simulink model "Hybrid_control"  (R2012b)
settings: Solver=ode3  StartTime=0.0  StopTime=inf  FixedStep=0.01  RelTol=1e-3
undefined symbols (not defined in the file or in its folder): HIL
libraries: quarc_library x7, simulink x1
settings Model: SimulationMode=external  ExtModeTrigDuration=5000  Creator=yiwei.liu  LastModifiedBy=yiwei.liu
settings SolverCC: PositivePriorityOrder=on
settings RTWCC: SystemTargetFile=quarc_win64.tlc  TemplateMakefile=quarc_default_tmf  Description=QUARC Win64 Target  ProcessScript=quarc_win64_make_rtw_hook
settings STFCustomTargetCC: TargetPreCompLibLocation=C:\PROGRA~3\QUARC\lib\2012b\win64\release  CodeReplacementLibrary=ANSI_C  GeneratePreprocessorConditionals=Disable all  CombineOutputUpdateFcns=on  GRTInterface=off  SystemTargetFile=quarc_win64.tlc
settings GRTTargetCC: TargetPreCompLibLocation=C:\PROGRA~3\QUARC\lib\2012b\win64\release  ParMdlRefBuildCompliant=off  CompOptLevelCompliant=off  ConcurrentExecutionCompliant=off  MatFileLogging=off  ExtMode=on  ExtModeMexFile=quarc_comm

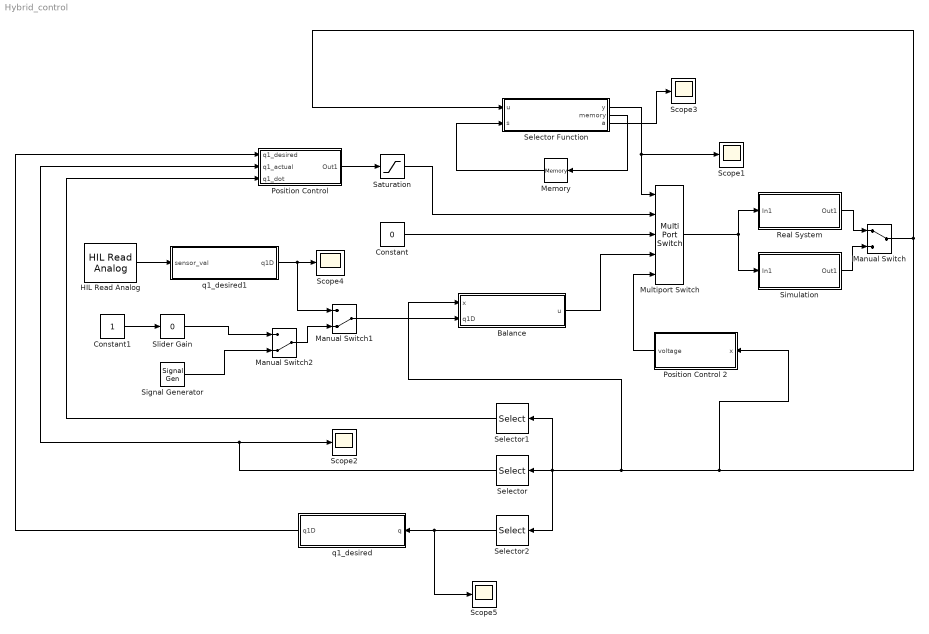
== system Hybrid_control ==
  Balance : MATLAB Function  TreatAsAtomicUnit=on
  Constant : Constant  Value=0
  Constant1 : Constant
  HIL Read Analog : quarc_library/Data Acquisition/Generic/Immediate I//O/HIL Read Analog  object_name=HIL-1  channels=[1]  sample_time=qc_get_step_size  active=on  vector_output=off
  Manual Switch : ManualSwitch
  Manual Switch1 : ManualSwitch  CurrentSetting=0
  Manual Switch2 : ManualSwitch  CurrentSetting=0
  Memory : Memory  X0=4
  Multiport Switch : MultiPortSwitch  Inputs=4
  Position Control : Subsystem  Tag=Simulation  Description=Simulation
  Position Control 2 : Subsystem  Tag=Simulation  Description=Simulation
  Real System : Subsystem
  Saturation : Saturate  UpperLimit=10  LowerLimit=-10
  Scope{1..5} (5 alike) : Scope
      Scope1 settings: TimeRange=10  YMin=3.8  YMax=4.2  SaveName=ScopeData3
      Scope2 settings: SaveName=ScopeData2
      Scope3 settings: YMin=2  YMax=2  SaveName=ScopeData4
      Scope4 settings: TimeRange=10  YMin=-3.5  YMax=5.5  SaveName=ScopeData5
      Scope5 settings: YMin=-12  YMax=9  SaveName=ScopeData6
  Selector : Selector  InputPortWidth=4  IndexOptions=Index vector (dialog)  Indices=[1]  OutputSizes=1
  Selector Function : MATLAB Function  TreatAsAtomicUnit=on
  Selector1 : Selector  InputPortWidth=4  IndexOptions=Index vector (dialog)  Indices=[2]  OutputSizes=1
  Selector2 : Selector  InputPortWidth=4  IndexOptions=Index vector (dialog)  Indices=[3,4]  OutputSizes=1
  Signal Generator : SignalGenerator  Frequency=0.5
  Simulation : Subsystem  Tag=Simulation  Description=Simulation
  Slider Gain : simulink/Math Operations/Slider Gain  low=-3.1416  gain=0  high=3.1416
  q1_desired : MATLAB Function  TreatAsAtomicUnit=on
  q1_desired1 : MATLAB Function  TreatAsAtomicUnit=on
  wires:
  Selector Function/1(y) -> Scope1/1, Multiport Switch/1
  Constant/1 -> Multiport Switch/3
  Selector Function/2(memory) -> Memory/1
  Simulation/1(Out1) -> Manual Switch/2
  Multiport Switch/1 -> Real System/1(In1), Simulation/1(In1)
  Real System/1(Out1) -> Manual Switch/1
  Manual Switch/1 -> Position Control 2/1(x), Balance/1(x), Selector1/1, Selector/1, Selector2/1, Selector Function/1(u)
  Memory/1 -> Selector Function/2(s)
  Position Control/1(Out1) -> Saturation/1
  Selector/1 -> Scope2/1, Position Control/2(q1_actual)
  Balance/1(u) -> Multiport Switch/4
  Selector1/1 -> Position Control/3(q1_dot)
  Selector2/1 -> Scope5/1, q1_desired/1(q)
  q1_desired/1(q1D) -> Position Control/1(q1_desired)
  Saturation/1 -> Multiport Switch/2
  Constant1/1 -> Slider Gain/1
  Position Control 2/1(voltage) -> Multiport Switch/5
  Selector Function/3(a) -> Scope3/1
  HIL Read Analog/1 -> q1_desired1/1(sensor_val)
  q1_desired1/1(q1D) -> Manual Switch1/1, Scope4/1
  Slider Gain/1 -> Manual Switch2/1
  Manual Switch1/1 -> Balance/2(q1D)
  Signal Generator/1 -> Manual Switch2/2
  Manual Switch2/1 -> Manual Switch1/2

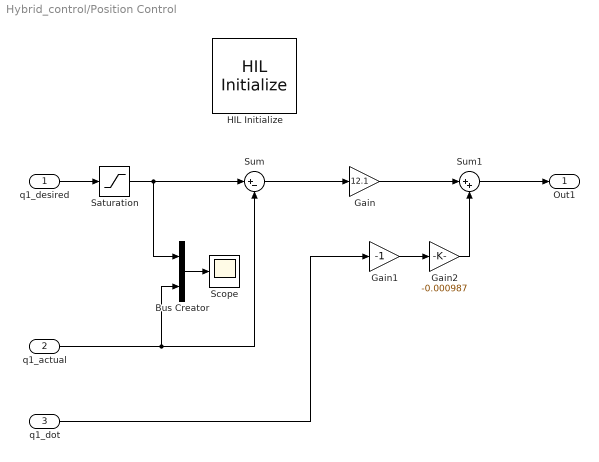
== system Hybrid_control/Position Control ==
  q1_desired : Inport  Description=q1 Desired
  q1_actual : Inport  Port=2
  q1_dot : Inport  Port=3
  Bus Creator : BusCreator  Inputs=2
  Gain : Gain  Gain=12.1
  Gain1 : Gain  Gain=-1
  Gain2 : Gain  Gain=-0.000987
  HIL Initialize : quarc_library/Data Acquisition/Generic/Configuration/HIL Initialize  Priority=-99  object_name=HIL-2  board_type=q2_usb  board_number=0  board_options=d0=digital;d1=digital;led=auto;update_rate=normal;decimation=1  exclusive=off  active=off  hardware_clocks=[0]  clock_modes=[]  initial_clock_frequencies=[]  set_clock_params_at_start=off  set_clock_params_at_switch_in=off  set_clock_frequencies_at_start=off  set_clock_frequencies_at_switch_in=off  analog_input_channels=[0:1]  analog_input_maximums=10  analog_input_minimums=-10  set_analog_input_params_at_start=on  set_analog_input_params_at_switch_in=off  analog_output_channels=[0:1]  analog_output_maximums=10  analog_output_minimums=-10  initial_analog_outputs=[0]  final_analog_outputs=[0]  watchdog_analog_outputs=0  set_analog_output_params_at_start=on  set_analog_output_params_at_switch_in=off  set_analog_outputs_at_start=on  set_analog_outputs_at_switch_in=off  set_analog_outputs_at_terminate=on  set_analog_outputs_at_switch_out=off  set_analog_outputs_on_watchdog=off  digital_input_channels=[]  digital_output_channels=[]  digital_output_configuration=[]  initial_digital_outputs=[1]  final_digital_outputs=[1]  watchdog_digital_outputs=[1]  set_digital_output_params_at_start=off  set_digital_output_params_at_switch_in=off  set_digital_outputs_at_start=on  set_digital_outputs_at_switch_in=off  set_digital_outputs_at_terminate=on  set_digital_outputs_at_switch_out=off  set_digital_outputs_on_watchdog=off  encoder_channels=[0:1]  quadrature=[4]  encoder_filter_frequency=[]  initial_encoder_counts=[0]  set_encoder_params_at_start=on  set_encoder_params_at_switch_in=off  set_encoder_counts_at_start=on  set_encoder_counts_at_switch_in=off  pwm_channels=[]  pwm_modes=[0]  pwm_frequency=1/0.020  pwm_configuration=[]  pwm_alignment=[]  pwm_polarity=[]  pwm_leading_deadband=[]  pwm_trailing_deadband=[]  initial_pwm_outputs=[0]  final_pwm_outputs=[0]  watchdog_pwm_outputs=[0]  set_pwm_params_at_start=on  set_pwm_params_at_switch_in=off  set_pwm_outputs_at_start=on  set_pwm_outputs_at_switch_in=off  set_pwm_outputs_at_terminate=on  set_pwm_outputs_at_switch_out=off  set_pwm_outputs_on_watchdog=off  other_output_channels=[]  initial_other_outputs=[]  final_other_outputs=[]  watchdog_other_outputs=[]  set_other_outputs_at_start=off  set_other_outputs_at_switch_in=off  set_other_outputs_at_terminate=off  set_other_outputs_at_switch_out=off  set_other_outputs_on_watchdog=off
  Saturation : Saturate  UpperLimit=pi/7  LowerLimit=-pi/7
  Scope : Scope
      settings: YMin=0.4  YMax=1.4
  Sum : Sum  Inputs=|+-
  Sum1 : Sum  Inputs=|++
  Out1 : Outport
  wires:
  Gain/1 -> Sum1/1
  Sum/1 -> Gain/1
  Gain1/1 -> Gain2/1
  Gain2/1 -> Sum1/2
  Bus Creator/1 -> Scope/1
  q1_desired/1 -> Saturation/1
  Sum1/1 -> Out1/1
  q1_actual/1 -> Bus Creator/2, Sum/2
  q1_dot/1 -> Gain1/1
  Saturation/1 -> Bus Creator/1, Sum/1

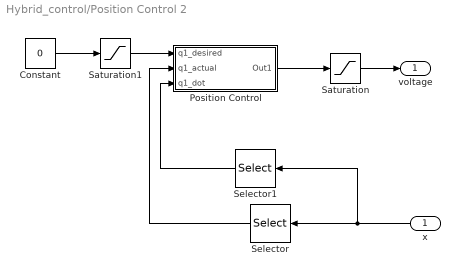
== system Hybrid_control/Position Control 2 ==
  x : Inport  Description=q1 Desired
  Constant : Constant  Value=0
  Position Control : Subsystem  Tag=Simulation  Description=Simulation
  Saturation : Saturate  UpperLimit=2  LowerLimit=-2
  Saturation1 : Saturate  UpperLimit=pi/6  LowerLimit=-pi/6
  Selector : Selector  InputPortWidth=4  IndexOptions=Index vector (dialog)  Indices=[1]  OutputSizes=1
  Selector1 : Selector  InputPortWidth=4  IndexOptions=Index vector (dialog)  Indices=[2]  OutputSizes=1
  voltage : Outport
  wires:
  Position Control/1(Out1) -> Saturation/1
  Selector/1 -> Position Control/2(q1_actual)
  Selector1/1 -> Position Control/3(q1_dot)
  Constant/1 -> Saturation1/1
  Saturation/1 -> voltage/1
  x/1 -> Selector1/1, Selector/1
  Saturation1/1 -> Position Control/1(q1_desired)

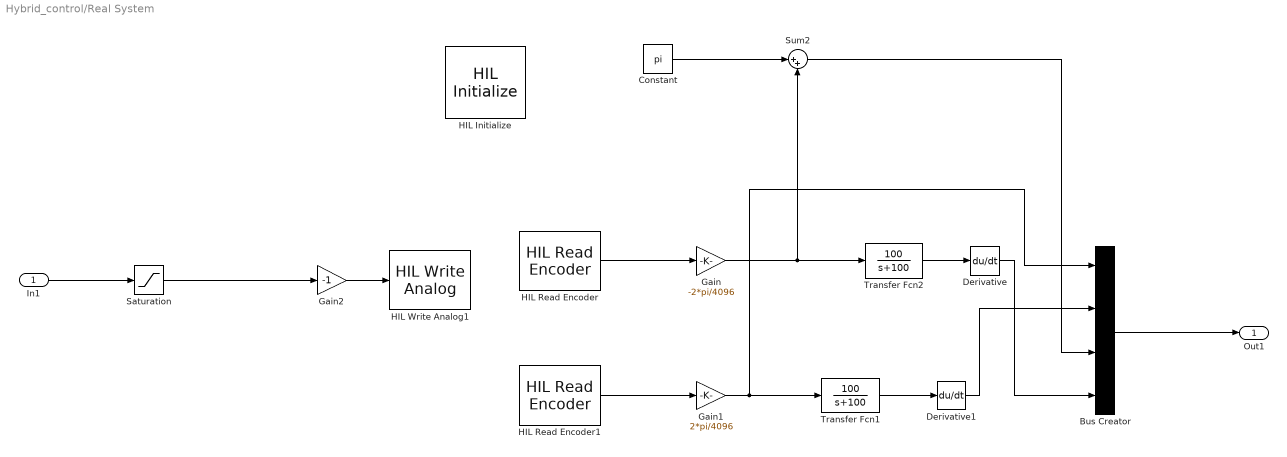
== system Hybrid_control/Real System ==
  In1 : Inport
  Bus Creator : BusCreator
  Constant : Constant  Value=pi
  Derivative : Derivative
  Derivative1 : Derivative
  Gain : Gain  Gain=-2*pi/4096
  Gain1 : Gain  Gain=2*pi/4096
  Gain2 : Gain  Gain=-1
  HIL Initialize : quarc_library/Data Acquisition/Generic/Configuration/HIL Initialize  Priority=-99  object_name=HIL-1  board_type=q2_usb  board_number=0  board_options=d0=digital;d1=digital;led=auto;update_rate=normal;decimation=1  exclusive=off  active=off  hardware_clocks=[0]  clock_modes=[]  initial_clock_frequencies=[]  set_clock_params_at_start=off  set_clock_params_at_switch_in=off  set_clock_frequencies_at_start=off  set_clock_frequencies_at_switch_in=off  analog_input_channels=[0:1]  analog_input_maximums=10  analog_input_minimums=-10  set_analog_input_params_at_start=on  set_analog_input_params_at_switch_in=off  analog_output_channels=[0:1]  analog_output_maximums=10  analog_output_minimums=-10  initial_analog_outputs=[0]  final_analog_outputs=[0]  watchdog_analog_outputs=0  set_analog_output_params_at_start=on  set_analog_output_params_at_switch_in=off  set_analog_outputs_at_start=on  set_analog_outputs_at_switch_in=off  set_analog_outputs_at_terminate=on  set_analog_outputs_at_switch_out=off  set_analog_outputs_on_watchdog=off  digital_input_channels=[]  digital_output_channels=[]  digital_output_configuration=[]  initial_digital_outputs=[1]  final_digital_outputs=[1]  watchdog_digital_outputs=[1]  set_digital_output_params_at_start=off  set_digital_output_params_at_switch_in=off  set_digital_outputs_at_start=on  set_digital_outputs_at_switch_in=off  set_digital_outputs_at_terminate=on  set_digital_outputs_at_switch_out=off  set_digital_outputs_on_watchdog=off  encoder_channels=[0:1]  quadrature=[4]  encoder_filter_frequency=[]  initial_encoder_counts=[0]  set_encoder_params_at_start=on  set_encoder_params_at_switch_in=off  set_encoder_counts_at_start=on  set_encoder_counts_at_switch_in=off  pwm_channels=[]  pwm_modes=[0]  pwm_frequency=1/0.020  pwm_configuration=[]  pwm_alignment=[]  pwm_polarity=[]  pwm_leading_deadband=[]  pwm_trailing_deadband=[]  initial_pwm_outputs=[0]  final_pwm_outputs=[0]  watchdog_pwm_outputs=[0]  set_pwm_params_at_start=on  set_pwm_params_at_switch_in=off  set_pwm_outputs_at_start=on  set_pwm_outputs_at_switch_in=off  set_pwm_outputs_at_terminate=on  set_pwm_outputs_at_switch_out=off  set_pwm_outputs_on_watchdog=off  other_output_channels=[]  initial_other_outputs=[]  final_other_outputs=[]  watchdog_other_outputs=[]  set_other_outputs_at_start=off  set_other_outputs_at_switch_in=off  set_other_outputs_at_terminate=off  set_other_outputs_at_switch_out=off  set_other_outputs_on_watchdog=off
  HIL Read Encoder : quarc_library/Data Acquisition/Generic/Immediate I//O/HIL Read Encoder  object_name=HIL-1  channels=[1]  sample_time=qc_get_step_size  active=on  vector_output=off  data_type_mode=Inherit via back propagation  data_type=double
  HIL Read Encoder1 : quarc_library/Data Acquisition/Generic/Immediate I//O/HIL Read Encoder  object_name=HIL-1  channels=[0]  sample_time=qc_get_step_size  active=on  vector_output=off  data_type_mode=Inherit via back propagation  data_type=double
  HIL Write Analog1 : quarc_library/Data Acquisition/Generic/Immediate I//O/HIL Write Analog  object_name=HIL-1  channels=0  sample_time=-1  active=off  vector_input=off
  Saturation : Saturate  UpperLimit=10  LowerLimit=-10
  Sum2 : Sum  Inputs=|++
  Transfer Fcn1 : TransferFcn  Numerator=[100]  Denominator=[1 100]
  Transfer Fcn2 : TransferFcn  Numerator=[100]  Denominator=[1 100]
  Out1 : Outport
  wires:
  Gain1/1 -> Transfer Fcn1/1, Bus Creator/1
  Bus Creator/1 -> Out1/1
  Derivative/1 -> Bus Creator/4
  Derivative1/1 -> Bus Creator/2
  Transfer Fcn1/1 -> Derivative1/1
  Saturation/1 -> Gain2/1
  HIL Read Encoder/1 -> Gain/1
  Gain/1 -> Transfer Fcn2/1, Sum2/2
  Gain2/1 -> HIL Write Analog1/1
  HIL Read Encoder1/1 -> Gain1/1
  Transfer Fcn2/1 -> Derivative/1
  Constant/1 -> Sum2/1
  Sum2/1 -> Bus Creator/3
  In1/1 -> Saturation/1

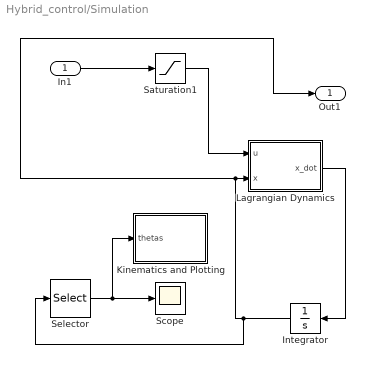
== system Hybrid_control/Simulation ==
  In1 : Inport
  Integrator : Integrator  InitialCondition=[0;0;pi-0.1;0]
  Kinematics and Plotting : MATLAB Function  TreatAsAtomicUnit=on
  Lagrangian Dynamics : MATLAB Function  TreatAsAtomicUnit=on
  Saturation1 : Saturate  UpperLimit=10  LowerLimit=-10
  Scope : Scope
      settings: YMin=-0.25  YMax=5.25
  Selector : Selector  InputPortWidth=4  IndexOptions=Index vector (dialog)  Indices=[1 3]  OutputSizes=1
  Out1 : Outport
  wires:
  Lagrangian Dynamics/1(x_dot) -> Integrator/1
  Integrator/1 -> Out1/1, Lagrangian Dynamics/2(x), Selector/1
  Selector/1 -> Kinematics and Plotting/1(thetas), Scope/1
  Saturation1/1 -> Lagrangian Dynamics/1(u)
  In1/1 -> Saturation1/1

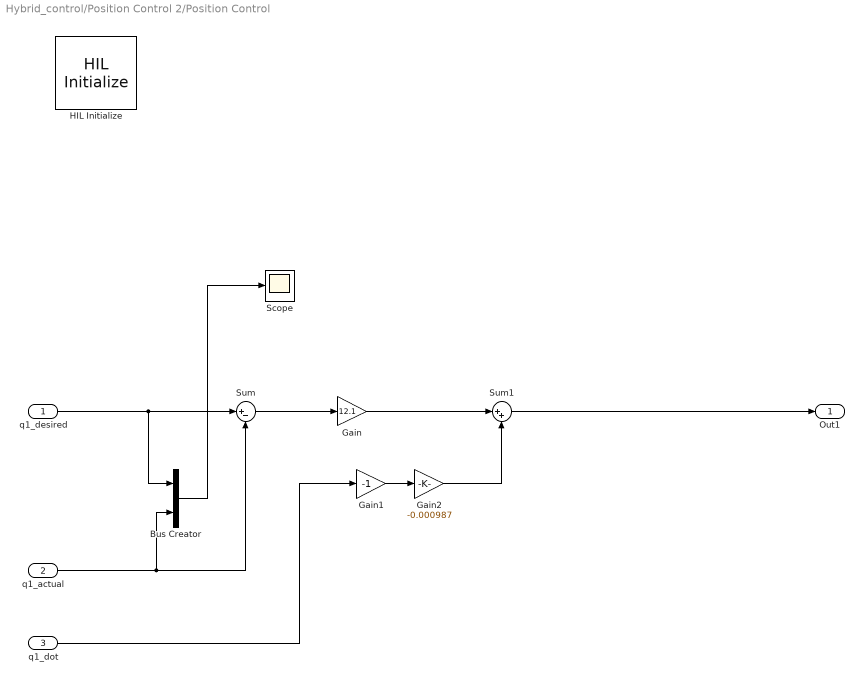
== system Hybrid_control/Position Control 2/Position Control ==
  q1_desired : Inport  Description=q1 Desired
  q1_actual : Inport  Port=2
  q1_dot : Inport  Port=3
  Bus Creator : BusCreator  Inputs=2
  Gain : Gain  Gain=12.1
  Gain1 : Gain  Gain=-1
  Gain2 : Gain  Gain=-0.000987
  HIL Initialize : quarc_library/Data Acquisition/Generic/Configuration/HIL Initialize  Priority=-99  object_name=HIL-3  board_type=q2_usb  board_number=0  board_options=d0=digital;d1=digital;led=auto;update_rate=normal;decimation=1  exclusive=off  active=off  hardware_clocks=[0]  clock_modes=[]  initial_clock_frequencies=[]  set_clock_params_at_start=off  set_clock_params_at_switch_in=off  set_clock_frequencies_at_start=off  set_clock_frequencies_at_switch_in=off  analog_input_channels=[0:1]  analog_input_maximums=10  analog_input_minimums=-10  set_analog_input_params_at_start=on  set_analog_input_params_at_switch_in=off  analog_output_channels=[0:1]  analog_output_maximums=10  analog_output_minimums=-10  initial_analog_outputs=[0]  final_analog_outputs=[0]  watchdog_analog_outputs=0  set_analog_output_params_at_start=on  set_analog_output_params_at_switch_in=off  set_analog_outputs_at_start=on  set_analog_outputs_at_switch_in=off  set_analog_outputs_at_terminate=on  set_analog_outputs_at_switch_out=off  set_analog_outputs_on_watchdog=off  digital_input_channels=[]  digital_output_channels=[]  digital_output_configuration=[]  initial_digital_outputs=[1]  final_digital_outputs=[1]  watchdog_digital_outputs=[1]  set_digital_output_params_at_start=off  set_digital_output_params_at_switch_in=off  set_digital_outputs_at_start=on  set_digital_outputs_at_switch_in=off  set_digital_outputs_at_terminate=on  set_digital_outputs_at_switch_out=off  set_digital_outputs_on_watchdog=off  encoder_channels=[0:1]  quadrature=[4]  encoder_filter_frequency=[]  initial_encoder_counts=[0]  set_encoder_params_at_start=on  set_encoder_params_at_switch_in=off  set_encoder_counts_at_start=on  set_encoder_counts_at_switch_in=off  pwm_channels=[]  pwm_modes=[0]  pwm_frequency=1/0.020  pwm_configuration=[]  pwm_alignment=[]  pwm_polarity=[]  pwm_leading_deadband=[]  pwm_trailing_deadband=[]  initial_pwm_outputs=[0]  final_pwm_outputs=[0]  watchdog_pwm_outputs=[0]  set_pwm_params_at_start=on  set_pwm_params_at_switch_in=off  set_pwm_outputs_at_start=on  set_pwm_outputs_at_switch_in=off  set_pwm_outputs_at_terminate=on  set_pwm_outputs_at_switch_out=off  set_pwm_outputs_on_watchdog=off  other_output_channels=[]  initial_other_outputs=[]  final_other_outputs=[]  watchdog_other_outputs=[]  set_other_outputs_at_start=off  set_other_outputs_at_switch_in=off  set_other_outputs_at_terminate=off  set_other_outputs_at_switch_out=off  set_other_outputs_on_watchdog=off
  Scope : Scope
      settings: YMin=0.4  YMax=1.4
  Sum : Sum  Inputs=|+-
  Sum1 : Sum  Inputs=|++
  Out1 : Outport
  wires:
  Gain/1 -> Sum1/1
  Sum/1 -> Gain/1
  Gain1/1 -> Gain2/1
  Gain2/1 -> Sum1/2
  Bus Creator/1 -> Scope/1
  Sum1/1 -> Out1/1
  q1_actual/1 -> Bus Creator/2, Sum/2
  q1_dot/1 -> Gain1/1
  q1_desired/1 -> Bus Creator/1, Sum/1

== matlab function Hybrid_control/Simulation/Kinematics and Plotting ==
  data: thetas input
function  fcn(thetas)
%#codegen
A=[0 0 0 0 0];
B=[0 0 6 6 8];
C=[0 -1 -1 0 0];
D=[1 1 1 1 1];

A2=[0 0];
B2=[0 12];
C2=[0 0];
D2=[1 1];
L1=6;

L2=2;
%First Link

    theta1=thetas(1);
    theta2=thetas(2);
    newpoints=trans(theta1,A,B,C,D);
    p= (newpoints(1:1,1:5));

    q= (newpoints(2:2,1:5));

    r= (newpoints(3:3,1:5));
   % Second Link

    new2=trans2(theta2,L1,L2,A2,B2,C2,D2);
    %Frame 1 to frame 0
    x2= new2(1:1,1:2);
    y2= new2(2:2,1:2);
    z2= new2(3:3,1:2);

    new3 = trans(theta1,x2,y2,z2,D2);
    %ABC values of Link 2 in frame 0
    p2= (new3(1:1,1:2));

    q2= (new3(2:2,1:2));

    r2= (new3(3:3,1:2));
   
%     hold on;

    plot3(p,q,r,'-b*',p2,q2,r2,'-g*');
    axis([-15,15,-15,15,-15,15]);
    grid on;
end

== matlab function Hybrid_control/Selector Function ==
  data: u input; y output; s input; memory output; a output
function [y,memory,a] = fcn(u,s)
% #codegen

q1 = u(1);
q2 = u(3);
q2_dot = u(4);


rad = atan2(sin(q2),cos(q2));
angle = rad*180/pi;
angle_1 = 10*pi/180;


section_1 = (angle>=170 && angle<=180) ||(angle>=-180 && angle<=-170);
section_2 = (angle>25 && angle<170) || (angle<-25 && angle>-170);
section_3 = (angle<=25 && angle>=-25);
section_4 = (q1>=angle_1 || q1<=-angle_1);



prev_state = s;


if(section_1 && abs(q2_dot)<=0.01)
    if(prev_state == 4 )
        
            current_state = 1;
        a=1;
    else
        a=2;
            current_state = prev_state;
    end

        
elseif(section_2 && abs(q2_dot)>=0.1)
    if(prev_state == 3) 
        current_state = 2;
      a=3
    else
        current_state = prev_state;
        a=4
    end
    
elseif(section_3)
    if(prev_state == 1) 
        current_state = 3;
    a=5;
    else
        current_state = prev_state;
       a=6;
        
    end

    
elseif( section_4 && abs(q2_dot)<=0.2 )
     if(prev_state == 2)
        %%if(abs(q2_dot)< 3)
            current_state = 4;
          a=7;
     else
         a=8;
         current_state = prev_state;
     end
     
else
    a=9;
    current_state = prev_state;

    
end 

q2_dot
y=current_state;
memory = current_state;

== matlab function Hybrid_control/Simulation/Lagrangian Dynamics ==
  data: u input; x_dot output; x input
function x_dot = fcn(u,x)
%#codegen
 
theta1= 0.0785;
theta2= 0.0272;
theta3= 0.0238;
theta4= 0.1145;
theta5= 0.5436;
theta6= 0.0107;

q1 = x(1);
q1_dot = x(2);
q2 = x(3);
q2_dot = x(4);
 
v = [u ; 0];
A = [theta1+theta2*(sin(q2)^2), theta3*cos(q2) ; theta3*cos(q2), theta2];
B = [2*theta2*sin(q2)*cos(q2)*q2_dot, (-1)*theta3*sin(q2)*q2_dot; (-1)*theta2*sin(q2)*cos(q2)*q1_dot,  0];
C = [theta5*q1_dot ; theta6*q2_dot];
D = [0 ;(-1)*theta4*9.8*sin(q2)];
 
%q_dd = [0;0];
q_dd = (A^(-1))*((v - B*[q1_dot ; q2_dot] - C - D)) ;
q1_dd = q_dd(1);
q2_dd = q_dd(2);
x_dot = [q1_dot ;q1_dd ; q2_dot; q2_dd ];
 
end

== matlab function Hybrid_control/Balance ==
  data: x input; u output; q1D input
function u = fcn(x,q1D)
q1A = x(1);
q2 = x(3);

q2 = atan2(sin(q2),cos(q2));
x(3) = q2;
k = [-0.9825 -1.3165 -15.6590 -2.2058];
x(1)

x(1) = q1A-q1D;
x(1)
u = -k * x;

== matlab function Hybrid_control/q1_desired ==
  data: q input; q1D output
function q1D  = fcn(q)
q2 = q(1)-pi;
q2dot = q(2);
q2 = atan2(sin(q2),cos(q2));


q1D = q2 * 1 + 0 * q2dot;

== matlab function Hybrid_control/q1_desired1 ==
  data: sensor_val input; q1D output
function q1D  = fcn(sensor_val)

OldValue = sensor_val;
OldMin = -5.5;
OldMax = 5;
NewMax = pi;
NewMin = -pi;
NewValue = (((OldValue - OldMin) * (NewMax - NewMin)) / (OldMax - OldMin)) + NewMin;

q1D = NewValue;
